simulink model "W3P2_model"  (R2020a)
settings: Solver=VariableStepAuto  StartTime=0.0  StopTime=10.0  RelTol=1e-3
settings Model: Creator=avn19  LastModifiedBy=avn19

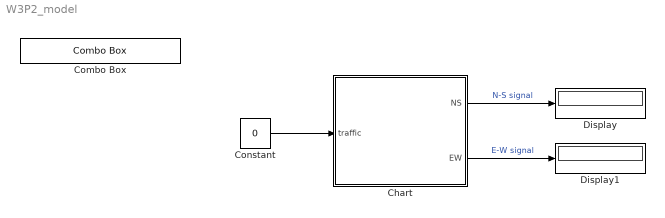
== system W3P2_model ==
  Chart : Stateflow chart  TreatAsAtomicUnit=on
  Combo Box : ComboBox  LabelPosition=Hide  SelectedLabel=Normal traffic
      settings: Values={{'Normal traffic', 'Traffic on North-South', 'Traffic on East-West'}, [0 1 2]}
  Constant : Constant  Value=0
  Display : Display
  Display1 : Display
  wires:
  Constant/1 -> Chart/1(traffic)
  Chart/1(NS) -> Display/1  "N-S signal"
  Chart/2(EW) -> Display1/1  "E-W signal"

== stateflow chart W3P2_model/Chart ==
  state stop
    NS = 1;
    EW= 3;
  state start_to_go
    NS = 2;
    EW = 1;
  state start_to_stop
    NS = 2;
    EW = 1;
  state go
    NS = 3;
    EW = 1;
  (default) -> stop
  stop -> start_to_go : [traffic == 0]{after(10,tick);}
  start_to_stop -> stop : [traffic == 0]
  start_to_go -> go : [traffic == 0]{after(3,tick);}
  go -> start_to_stop : [traffic == 0]{after(20,tick);}
  data: traffic input; NS output; EW output
